simulink model "task8_simulink_backup_semilineare"  (R2024b)
settings: Solver=VariableStepAuto  StartTime=0.0  StopTime=10.0  RelTol=1e-3
undefined symbols (not defined in the file): A, B, x_trim
settings Model: Creator=Admin  LastModifiedBy=Admin

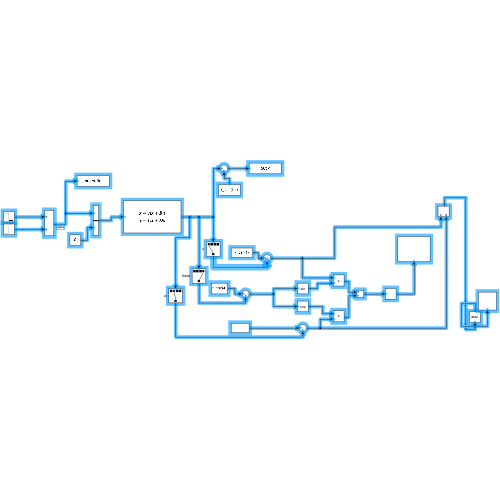
[thumbnail: Simulink's stored preview of the top-level diagram]
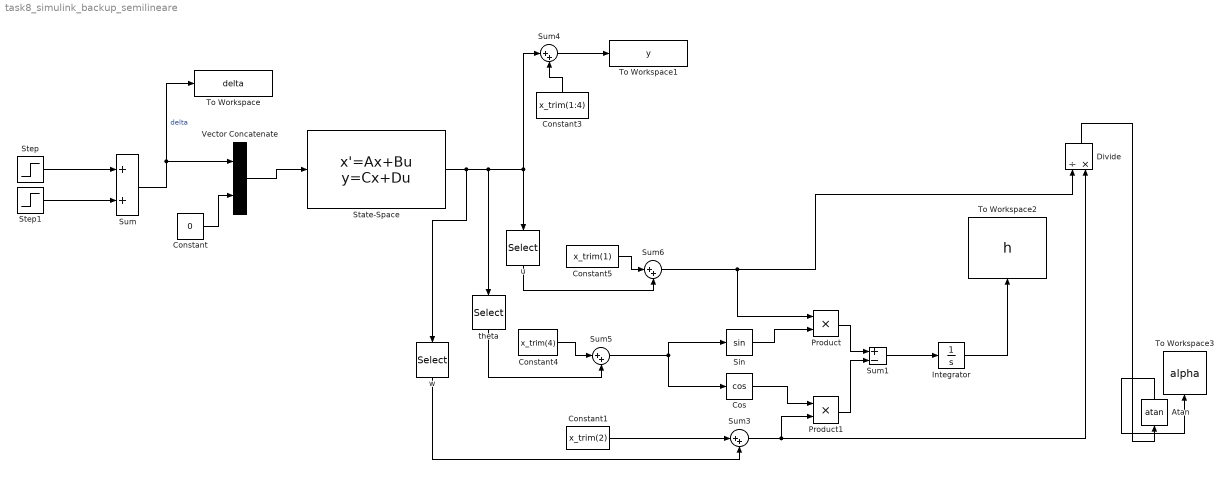
== system task8_simulink_backup_semilineare ==
  Atan : Trigonometry  Operator=atan
  Constant : Constant  Value=0
  Constant1 : Constant  Value=x_trim(2)
  Constant3 : Constant  Value=x_trim(1:4)
  Constant4 : Constant  Value=x_trim(4)
  Constant5 : Constant  Value=x_trim(1)
  Cos : Trigonometry  Operator=cos
  Divide : Product  Inputs=/*
  Integrator : Integrator
  Product : Product
  Product1 : Product
  Sin : Trigonometry
  State-Space : StateSpace  A=A  B=B  C=eye(4)  D=zeros(4,2)  InitialCondition=zeros(4,1)
  Step : Step  Time=5  After=- pi/180  SampleTime=0
  Step1 : Step  Time=10  After=(pi/180)  SampleTime=0
  Sum : Sum
  Sum1 : Sum  Inputs=+-
  Sum{3..6} (4 alike) : Sum  Inputs=|++
  To Workspace : ToWorkspace  VariableName=delta  SampleTime=-1
  To Workspace1 : ToWorkspace  VariableName=y  SaveFormat=Structure  SampleTime=-1
      settings: Save2DSignal=2-D array (concatenate along first dimension)
  To Workspace2 : ToWorkspace  VariableName=h  SampleTime=-1
      settings: Save2DSignal=2-D array (concatenate along first dimension)
  To Workspace3 : ToWorkspace  VariableName=alpha  SampleTime=-1
      settings: Save2DSignal=2-D array (concatenate along first dimension)
  Vector Concatenate : Concatenate
  theta : Selector  InputPortWidth=4  IndexOptions=Index vector (dialog)  Indices=4  OutputSizes=1
  u : Selector  InputPortWidth=4  IndexOptions=Index vector (dialog)  Indices=1  OutputSizes=1
  w : Selector  InputPortWidth=4  IndexOptions=Index vector (dialog)  Indices=2  OutputSizes=1
  wires:
  Product1/1 -> Sum1/2
  Atan/1 -> To Workspace3/1
  Sum4/1 -> To Workspace1/1
  Divide/1 -> Atan/1
  Sum1/1 -> Integrator/1
  theta/1 -> Sum5/2
  Constant4/1 -> Sum5/1
  Integrator/1 -> To Workspace2/1
  Constant5/1 -> Sum6/1
  Sum6/1 -> Divide/1, Product/1
  Cos/1 -> Product1/1
  Constant3/1 -> Sum4/2
  Product/1 -> Sum1/1
  Sin/1 -> Product/2
  Step/1 -> Sum/1
  Sum5/1 -> Cos/1, Sin/1
  Constant/1 -> Vector Concatenate/2
  Sum/1 -> Vector Concatenate/1, To Workspace/1  "delta"
  State-Space/1 -> theta/1, Sum4/1, u/1, w/1
  Sum3/1 -> Divide/2, Product1/2
  Vector Concatenate/1 -> State-Space/1
  Step1/1 -> Sum/2
  w/1 -> Sum3/2
  Constant1/1 -> Sum3/1
  u/1 -> Sum6/2
